simulink model "Fixed_transmission_ratio"  (R2022a)
settings: Solver=VariableStepAuto  StartTime=0.0  StopTime=10.0  RelTol=1e-3
model workspace (MAT data in the model file):
  CA = 2.77
  If = 0.218
  Iw1 = 1.798
  Iw2 = 3.598
  L = 3.2
  a = 1.947
  f = 0.013
  g = 9.8
  hg = 0.9
  i0 = 5.83
  j = 0
  kt = 0.85
  m1 = 1800
  m2 = 3880
  r = 0.367
libraries: simulink x1
settings Model: Creator=cht  LastModifiedBy=cht
settings DataIOCC: SaveFormat=Array  SaveOutput=off  InspectSignalLogs=on  SaveTime=off  ReturnWorkspaceOutputs=off

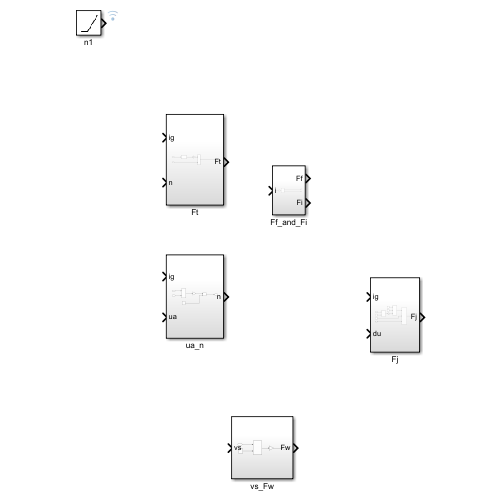
[thumbnail: Simulink's stored preview of the top-level diagram]
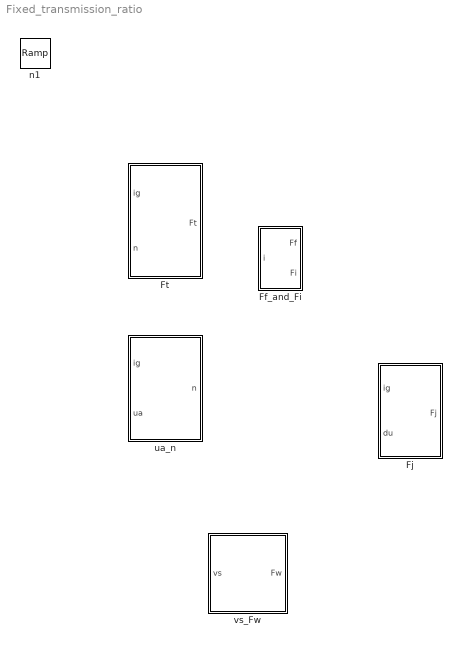
== system Fixed_transmission_ratio ==
  Ff_and_Fi : Subsystem
  Fj : Subsystem
  Ft : Subsystem
  n1 : simulink/Sources/Ramp  slope=340  start=0  InitialOutput=600
  ua_n : Subsystem
  vs_Fw : Subsystem

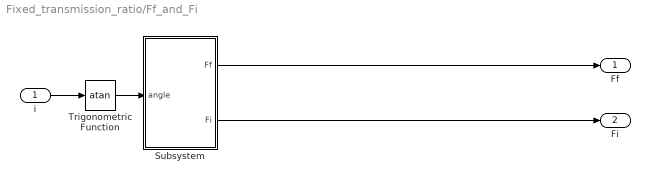
== system Fixed_transmission_ratio/Ff_and_Fi ==
  i : Inport
  Subsystem : Subsystem
  Trigonometric Function : Trigonometry  Operator=atan
  Ff : Outport
  Fi : Outport  Port=2
  wires:
  i/1 -> Trigonometric Function/1
  Subsystem/1(Ff) -> Ff/1
  Trigonometric Function/1 -> Subsystem/1(angle)
  Subsystem/2(Fi) -> Fi/1

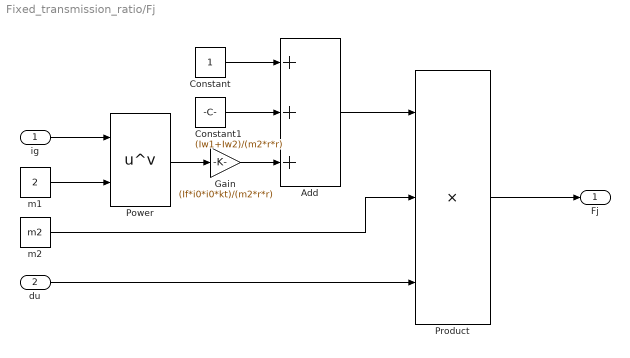
== system Fixed_transmission_ratio/Fj ==
  ig : Inport
  du : Inport  Port=2
  Add : Sum  Inputs=+++
  Constant : Constant
  Constant1 : Constant  Value=(Iw1+Iw2)/(m2*r*r)
  Gain : Gain  Gain=(If*i0*i0*kt)/(m2*r*r)
  Power : Math  Operator=pow
  Product : Product  Inputs=3
  m1 : Constant  Value=2
  m2 : Constant  Value=m2
  Fj : Outport
  wires:
  Constant1/1 -> Add/2
  Power/1 -> Gain/1
  Gain/1 -> Add/3
  Constant/1 -> Add/1
  du/1 -> Product/3
  ig/1 -> Power/1
  Product/1 -> Fj/1
  Add/1 -> Product/1
  m2/1 -> Product/2
  m1/1 -> Power/2

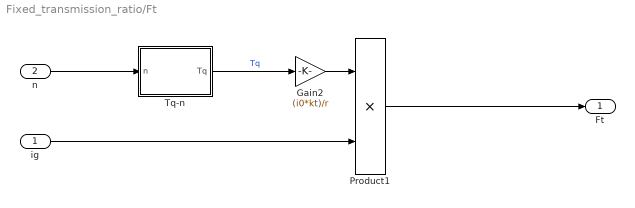
== system Fixed_transmission_ratio/Ft ==
  ig : Inport
  n : Inport  Port=2
  Gain2 : Gain  Gain=(i0*kt)/r
  Product1 : Product
  Tq-n : MATLAB Function  TreatAsAtomicUnit=on
  Ft : Outport
  wires:
  Product1/1 -> Ft/1
  ig/1 -> Product1/2
  Tq-n/1(Tq) -> Gain2/1  "Tq"
  n/1 -> Tq-n/1(n)
  Gain2/1 -> Product1/1

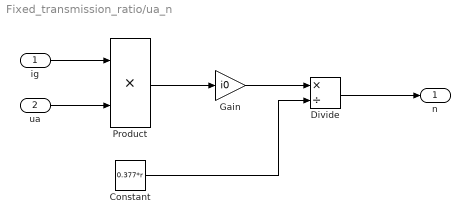
== system Fixed_transmission_ratio/ua_n ==
  ig : Inport
  ua : Inport  Port=2
  Constant : Constant  Value=0.377*r
  Divide : Product  Inputs=*/
  Gain : Gain  Gain=i0
  Product : Product
  n : Outport
  wires:
  ua/1 -> Product/2
  Product/1 -> Gain/1
  Divide/1 -> n/1
  Constant/1 -> Divide/2
  Gain/1 -> Divide/1
  ig/1 -> Product/1

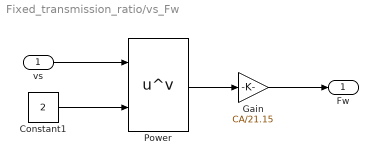
== system Fixed_transmission_ratio/vs_Fw ==
  vs : Inport
  Constant1 : Constant  Value=2
  Gain : Gain  Gain=CA/21.15
  Power : Math  Operator=pow
  Fw : Outport
  wires:
  Constant1/1 -> Power/2
  Gain/1 -> Fw/1
  vs/1 -> Power/1
  Power/1 -> Gain/1

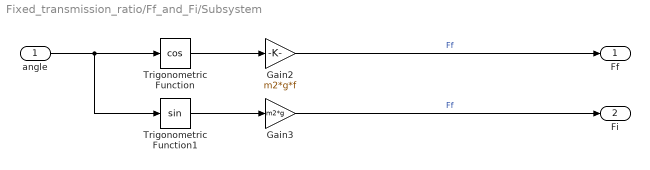
== system Fixed_transmission_ratio/Ff_and_Fi/Subsystem ==
  angle : Inport
  Gain2 : Gain  Gain=m2*g*f
  Gain3 : Gain  Gain=m2*g
  Trigonometric Function : Trigonometry  Operator=cos
  Trigonometric Function1 : Trigonometry
  Ff : Outport
  Fi : Outport  Port=2
  wires:
  Gain3/1 -> Fi/1  "Ff"
  angle/1 -> Trigonometric Function1/1, Trigonometric Function/1
  Trigonometric Function1/1 -> Gain3/1
  Trigonometric Function/1 -> Gain2/1
  Gain2/1 -> Ff/1  "Ff"

== matlab function Fixed_transmission_ratio/Ft/Tq-n ==
  data: n input; Tq output
function Tq = fcn(n)
%#codegen

Tq = -19.313+295.27*(n/1000)-165.44*(n/1000)^2+40.874*(n/1000)^3-3.8445*(n/1000)^4;
